simulink model "Main_Data_FlowAyush_V1"  (R2023b)
settings: Solver=FixedStepAuto  StartTime=0.0  StopTime=10.0  FixedStep=1e-3  RelTol=1e-3  EnableMultiTasking=on
undefined symbols (not defined in the file): D0, D1, D10, D11, D12, D13, D14, D15, D2, D3, D4, D5, D6, D7, D8, D9, PTA0, PTA1, PTA2, PTB23, PTB9, PTC16, PTC17, PTC2, PTC3, PTC4, PTD0, PTD1, PTD2, PTD3, PTE24, PTE25
libraries: frdmk64flib x16
settings Model: ExtModeTrigDuration=5  Creator=sadeg  LastModifiedBy=ayush
settings OptimizationCC: EnhancedBackFolding=on  PassReuseOutputArgsThreshold=0  MaxStackSize=64  OptimizeBlockOrder=speed  DifferentSizesBufferReuse=on  OptimizationCustomize=off
settings DebuggingCC: ParameterTunabilityLossMsg=error
settings HardwareCC: ProdBitPerPointer=32  ProdBitPerSizeT=32  ProdBitPerPtrDiffT=32  ProdLargestAtomicInteger=Long  ProdLargestAtomicFloat=Double  ProdWordSize=32  ProdHWDeviceType=ARM Compatible->ARM Cortex  UseEmbeddedCoderFeatures=off
settings SFSimCC: MATLABDynamicMemAlloc=off
settings RTWCC: Description=Embedded Coder  SystemTargetFile=ert.tlc  HardwareBoard=NXP FRDM-K64F  TLCOptions="-aInlineSetEventsForThisBaseRateFcn=TLC_FALSE -aSuppressMultiTaskScheduler=TLC_FALSE  -aRateBasedStepFcn=0"  TemplateMakefile=ert_default_tmf  Toolchain=GNU Tools for ARM Embedded Processors
settings CodeAppCC: ForceParamTrailComments=on  OperatorAnnotations=on
settings ERTTargetCC: ERTCustomFileBanners=off  SupportContinuousTime=on  SupportNonInlinedSFcns=on  RemoveResetFunc=off  ModelStepFunctionPrototypeControlCompliant=off  ExtModeTransport=4  ExtModeMexFile=sendToCommService

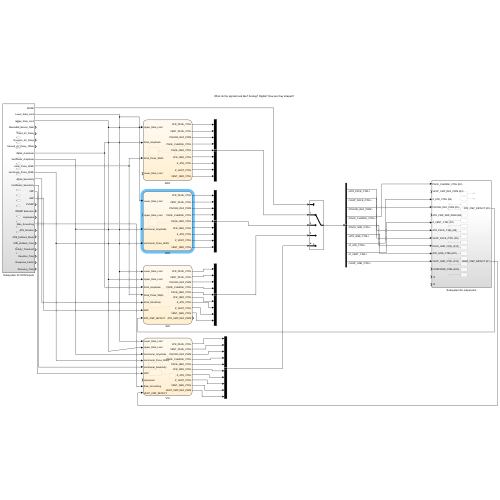
[thumbnail: Simulink's stored preview of the top-level diagram]
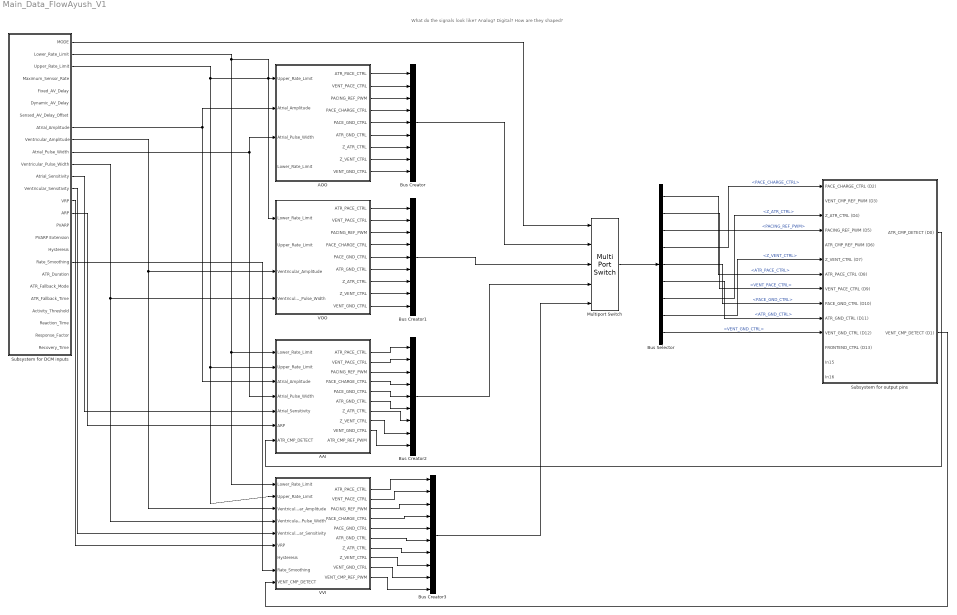
== system Main_Data_FlowAyush_V1 ==
  note: What do the signals look like? Analog? Digital? How are they shaped?
  AAI : Stateflow chart  TreatAsAtomicUnit=on
  AOO : Stateflow chart  TreatAsAtomicUnit=on
      settings: PortSchema="{\"entries\":[{\"content\":{\"sides\":[{\"content\":{\"connectorIds\":[\"In1\",\"In2\",\"In3\",\"In4\"]},\"type\":\"ConnectorPlacement.EquallySpacedRectSide\",\"uuid\":\"492a7fcf-0136-4cc6-a368-2e6eb8f4a8f6\"},{\"content\":{\"connectorIds\":[\"Out1\",\"Out2\",\"Out3\",\"Out4\",\"Out5\",\"Out8\",\"Out6\",\"Out7\",\"Out9\"],\"side\":\"RIGHT\"},\"type\":\"ConnectorPlacement.EquallySpacedRectSide\",\"uuid\":\"446f1639-51dc-43c3-8eec-8a39ae78ded7\"},{\"content\":{\"side\":\"TOP\"},\"type\":\"ConnectorPlacement.EquallySpacedRectSide\",\"uuid\":\"77fd6d12-343c-45d8-9399-9fe0379be2cf\"}]},\"type\":\"ConnectorPlacement.EquallySpacedConnector\",\"uuid\":\"42a5ffd8-4660-4821-97a9-3a811e8cbc3e\"}],\"packageUris\":[\"http://schema.mathworks.com/mf0/Connector/R2020b\"],\"version\":\"1.0\"}"
  Bus Creator : BusCreator  Inputs=9
  Bus Creator1 : BusCreator  Inputs=9
  Bus Creator2 : BusCreator  Inputs=9
  Bus Creator3 : BusCreator  Inputs=10
  Bus Selector : BusSelector  OutputSignals=ATR_PACE_CTRL,VENT_PACE_CTRL,PACING_REF_PWM,PACE_CHARGE_CTRL,PACE_GND_CTRL,ATR_GND_CTRL,Z_ATR_CTRL,Z_VENT_CTRL,VENT_GND_CTRL
  Multiport Switch : MultiPortSwitch  Inputs=4  SaturateOnIntegerOverflow=off  InputSameDT=off
  Subsystem for DCM inputs : Subsystem
  Subsystem for output pins : Subsystem
  VOO : Stateflow chart  TreatAsAtomicUnit=on
  VVI : Stateflow chart  TreatAsAtomicUnit=on
  wires:
  Subsystem for DCM inputs/2(Lower_Rate_Limit) -> VVI/1(Lower_Rate_Limit), AAI/1(Lower_Rate_Limit), VOO/1(Lower_Rate_Limit)
  Subsystem for DCM inputs/3(Upper_Rate_Limit) -> VVI/2(Upper_Rate_Limit), AAI/2(Upper_Rate_Limit), AOO/1(Upper_Rate_Limit)
  Subsystem for DCM inputs/8(Atrial_Amplitude) -> AAI/3(Atrial_Amplitude), AOO/2(Atrial_Amplitude)
  Subsystem for DCM inputs/10(Atrial_Pulse_Width) -> AAI/4(Atrial_Pulse_Width), AOO/3(Atrial_Pulse_Width)
  Subsystem for DCM inputs/9(Ventricular_Amplitude) -> VVI/3(Ventricular_Amplitude), VOO/3(Ventricular_Amplitude)
  Subsystem for DCM inputs/11(Ventricular_Pulse_Width) -> VVI/4(Ventricular_Pulse_Width), VOO/4(Ventricular_Pulse_Width)
  Subsystem for DCM inputs/12(Atrial_Sensitivity) -> AAI/5(Atrial_Sensitivity)
  Subsystem for DCM inputs/15(ARP) -> AAI/6(ARP)
  Subsystem for DCM inputs/19(Rate_Smoothing) -> VVI/8(Rate_Smoothing)
  Subsystem for DCM inputs/13(Ventricular_Sensitivity) -> VVI/5(Ventricular_Sensitivity)
  Subsystem for DCM inputs/14(VRP) -> VVI/6(VRP)
  AOO/1(ATR_PACE_CTRL) -> Bus Creator/1
  AOO/2(VENT_PACE_CTRL) -> Bus Creator/2
  AOO/3(PACING_REF_PWM) -> Bus Creator/3
  AOO/4(PACE_CHARGE_CTRL) -> Bus Creator/4
  AOO/5(PACE_GND_CTRL) -> Bus Creator/5
  AOO/8(ATR_GND_CTRL) -> Bus Creator/6
  AOO/6(Z_ATR_CTRL) -> Bus Creator/7
  AOO/7(Z_VENT_CTRL) -> Bus Creator/8
  AOO/9(VENT_GND_CTRL) -> Bus Creator/9
  VOO/1(ATR_PACE_CTRL) -> Bus Creator1/1
  VOO/2(VENT_PACE_CTRL) -> Bus Creator1/2
  VOO/3(PACING_REF_PWM) -> Bus Creator1/3
  VOO/4(PACE_CHARGE_CTRL) -> Bus Creator1/4
  VOO/5(PACE_GND_CTRL) -> Bus Creator1/5
  VOO/6(ATR_GND_CTRL) -> Bus Creator1/6
  VOO/7(Z_ATR_CTRL) -> Bus Creator1/7
  VOO/8(Z_VENT_CTRL) -> Bus Creator1/8
  VOO/9(VENT_GND_CTRL) -> Bus Creator1/9
  AAI/9(VENT_GND_CTRL) -> Bus Creator2/9
  AAI/2(VENT_PACE_CTRL) -> Bus Creator2/2
  AAI/1(ATR_PACE_CTRL) -> Bus Creator2/1
  AAI/4(PACE_CHARGE_CTRL) -> Bus Creator2/4
  AAI/6(ATR_GND_CTRL) -> Bus Creator2/6
  AAI/3(PACING_REF_PWM) -> Bus Creator2/3
  AAI/7(Z_ATR_CTRL) -> Bus Creator2/7
  AAI/8(Z_VENT_CTRL) -> Bus Creator2/8
  AAI/5(PACE_GND_CTRL) -> Bus Creator2/5
  VVI/9(VENT_GND_CTRL) -> Bus Creator3/9
  VVI/2(VENT_PACE_CTRL) -> Bus Creator3/2
  VVI/1(ATR_PACE_CTRL) -> Bus Creator3/1
  VVI/4(PACE_CHARGE_CTRL) -> Bus Creator3/4
  VVI/6(ATR_GND_CTRL) -> Bus Creator3/6
  VVI/3(PACING_REF_PWM) -> Bus Creator3/3
  VVI/7(Z_ATR_CTRL) -> Bus Creator3/7
  VVI/8(Z_VENT_CTRL) -> Bus Creator3/8
  VVI/5(PACE_GND_CTRL) -> Bus Creator3/5
  Multiport Switch/1 -> Bus Selector/1
  Bus Creator/1 -> Multiport Switch/2
  Bus Creator1/1 -> Multiport Switch/3
  Bus Creator2/1 -> Multiport Switch/4
  Bus Creator3/1 -> Multiport Switch/5
  Subsystem for DCM inputs/1(MODE) -> Multiport Switch/1
  Bus Selector/1 -> Subsystem for output pins/7(ATR_PACE_CTRL (D8))  "<ATR_PACE_CTRL>"
  Bus Selector/2 -> Subsystem for output pins/8(VENT_PACE_CTRL (D9))  "<VENT_PACE_CTRL>"
  Bus Selector/3 -> Subsystem for output pins/4(PACING_REF_PWM (D5))  "<PACING_REF_PWM>"
  Bus Selector/4 -> Subsystem for output pins/1(PACE_CHARGE_CTRL (D2))  "<PACE_CHARGE_CTRL>"
  Bus Selector/5 -> Subsystem for output pins/9(PACE_GND_CTRL (D10))  "<PACE_GND_CTRL>"
  Bus Selector/6 -> Subsystem for output pins/10(ATR_GND_CTRL (D11))  "<ATR_GND_CTRL>"
  Bus Selector/7 -> Subsystem for output pins/3(Z_ATR_CTRL (D4))  "<Z_ATR_CTRL>"
  Bus Selector/8 -> Subsystem for output pins/6(Z_VENT_CTRL (D7))  "<Z_VENT_CTRL>"
  Bus Selector/9 -> Subsystem for output pins/11(VENT_GND_CTRL (D12))  "<VENT_GND_CTRL>"
  VVI/10(VENT_CMP_REF_PWM) -> Bus Creator3/10
  Subsystem for output pins/2(VENT_CMP_DETECT (D1)) -> VVI/9(VENT_CMP_DETECT)
  Subsystem for output pins/1(ATR_CMP_DETECT (D0)) -> AAI/7(ATR_CMP_DETECT)

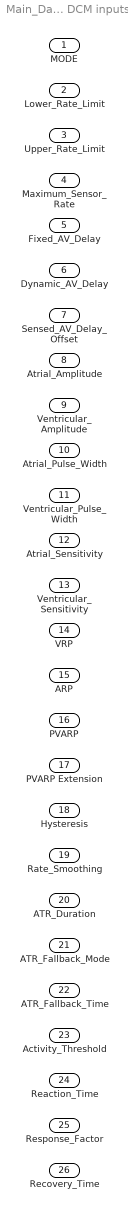
== system Main_Data_FlowAyush_V1/Subsystem for DCM inputs ==
  MODE : Outport
  Lower_Rate_Limit : Outport  Port=2
  Upper_Rate_Limit : Outport  Port=3
  Maximum_Sensor_Rate : Outport  Port=4
  Fixed_AV_Delay : Outport  Port=5
  Dynamic_AV_Delay : Outport  Port=6
  Sensed_AV_Delay_Offset : Outport  Port=7
  Atrial_Amplitude : Outport  Port=8
  Ventricular_Amplitude : Outport  Port=9
  Atrial_Pulse_Width : Outport  Port=10
  Ventricular_Pulse_Width : Outport  Port=11
  Atrial_Sensitivity : Outport  Port=12
  Ventricular_Sensitivity : Outport  Port=13
  VRP : Outport  Port=14
  ARP : Outport  Port=15
  PVARP : Outport  Port=16
  PVARP Extension : Outport  Port=17
  Hysteresis : Outport  Port=18
  Rate_Smoothing : Outport  Port=19
  ATR_Duration : Outport  Port=20
  ATR_Fallback_Mode : Outport  Port=21
  ATR_Fallback_Time : Outport  Port=22
  Activity_Threshold : Outport  Port=23
  Reaction_Time : Outport  Port=24
  Response_Factor : Outport  Port=25
  Recovery_Time : Outport  Port=26

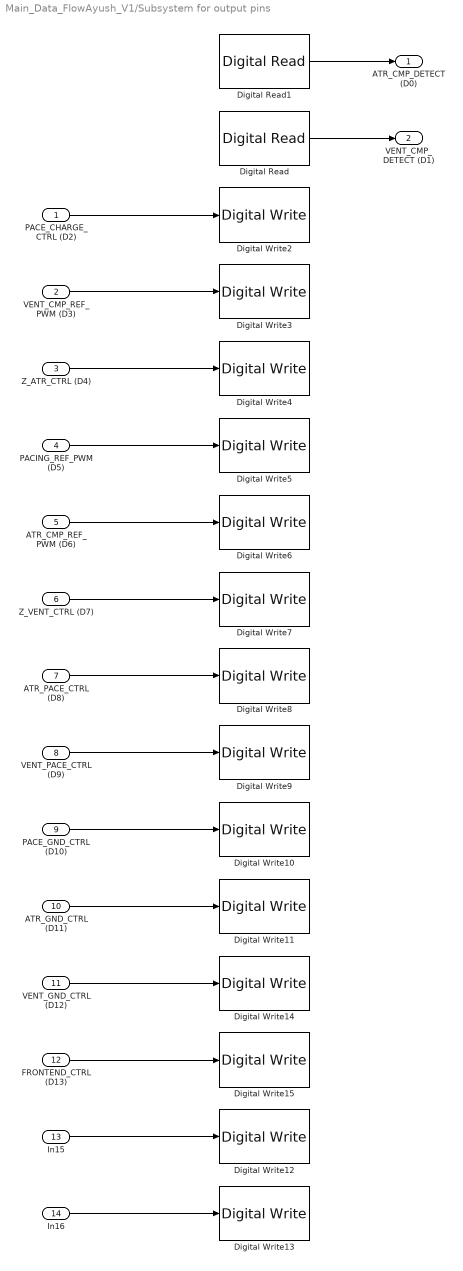
== system Main_Data_FlowAyush_V1/Subsystem for output pins ==
  PACE_CHARGE_CTRL (D2) : Inport
  VENT_CMP_REF_PWM (D3) : Inport  Port=2
  Z_ATR_CTRL (D4) : Inport  Port=3
  PACING_REF_PWM (D5) : Inport  Port=4
  ATR_CMP_REF_PWM (D6) : Inport  Port=5
  Z_VENT_CTRL (D7) : Inport  Port=6
  ATR_PACE_CTRL (D8) : Inport  Port=7
  VENT_PACE_CTRL (D9) : Inport  Port=8
  PACE_GND_CTRL (D10) : Inport  Port=9
  ATR_GND_CTRL (D11) : Inport  Port=10
  VENT_GND_CTRL (D12) : Inport  Port=11
  FRONTEND_CTRL (D13) : Inport  Port=12
  In15 : Inport  Port=13
  In16 : Inport  Port=14
  Digital Read : frdmk64flib/Digital Read  Whichpin=PTC17 (D1)  SampleTime=-1
  Digital Read1 : frdmk64flib/Digital Read  Whichpin=PTC16 (D0)  SampleTime=-1
  Digital Write10 : frdmk64flib/Digital Write  Whichpin=PTD0 (D10)
  Digital Write11 : frdmk64flib/Digital Write  Whichpin=PTD2 (D11)
  Digital Write12 : frdmk64flib/Digital Write  Whichpin=PTE25 (D14)
  Digital Write13 : frdmk64flib/Digital Write  Whichpin=PTE24 (D15)
  Digital Write14 : frdmk64flib/Digital Write  Whichpin=PTD3 (D12)
  Digital Write15 : frdmk64flib/Digital Write  Whichpin=PTD1 (D13)
  Digital Write2 : frdmk64flib/Digital Write  Whichpin=PTB9 (D2)
  Digital Write3 : frdmk64flib/Digital Write  Whichpin=PTA1 (D3)
  Digital Write4 : frdmk64flib/Digital Write  Whichpin=PTB23 (D4)
  Digital Write5 : frdmk64flib/Digital Write  Whichpin=PTA2 (D5)
  Digital Write6 : frdmk64flib/Digital Write  Whichpin=PTC2 (D6)
  Digital Write7 : frdmk64flib/Digital Write  Whichpin=PTC3 (D7)
  Digital Write8 : frdmk64flib/Digital Write  Whichpin=PTA0 (D8)
  Digital Write9 : frdmk64flib/Digital Write  Whichpin=PTC4 (D9)
  ATR_CMP_DETECT (D0) : Outport
  VENT_CMP_DETECT (D1) : Outport  Port=2
  wires:
  PACE_CHARGE_CTRL (D2)/1 -> Digital Write2/1
  Z_ATR_CTRL (D4)/1 -> Digital Write4/1
  VENT_CMP_REF_PWM (D3)/1 -> Digital Write3/1
  PACING_REF_PWM (D5)/1 -> Digital Write5/1
  Z_VENT_CTRL (D7)/1 -> Digital Write7/1
  ATR_CMP_REF_PWM (D6)/1 -> Digital Write6/1
  PACE_GND_CTRL (D10)/1 -> Digital Write10/1
  ATR_GND_CTRL (D11)/1 -> Digital Write11/1
  ATR_PACE_CTRL (D8)/1 -> Digital Write8/1
  VENT_PACE_CTRL (D9)/1 -> Digital Write9/1
  In15/1 -> Digital Write12/1
  VENT_GND_CTRL (D12)/1 -> Digital Write14/1
  FRONTEND_CTRL (D13)/1 -> Digital Write15/1
  In16/1 -> Digital Write13/1
  Digital Read/1 -> VENT_CMP_DETECT (D1)/1
  Digital Read1/1 -> ATR_CMP_DETECT (D0)/1

== stateflow chart Main_Data_FlowAyush_V1/AOO ==
  note: AOO: Pace Atrium at constant rate
  state DISCHARGE
    during:
    %Discharge C22 into Atrium
    %Begin Charging C21 Blocking Capacitor
    PACE_CHARGE_CTRL = 0;
    PACE_GND_CTRL = 1;
    ATR_PACE_CTRL = 1;
    ATR_GND_CTRL = 0;
    Z_ATR_CTRL = 0;
    Z_VENT_CTRL = 0;
    VENT_GND_CTRL = 0;
    VENT_PACE_CTRL  = 0;
  state CHARGE
    during:
    % Start Charging C22
    ATR_PACE_CTRL = 0;
    VENT_PACE_CTRL = 0;
    PACING_REF_PWM = Atrial_Amplitude
    PACE_CHARGE_CTRL = 1;
    %Begin Discharging C21 Blocking Capacitor
    PACE_GND_CTRL = 1;
    VENT_PACE_CTRL = 0;
    VENT_GND_CTRL = 0;
    Z_ATR_CTRL = 0;
    Z_VENT_CTRL = 0;
    ATR_PACE_CTRL = 0;
    ATR_GND_CTRL = 1;
  (default) -> CHARGE
  CHARGE -> DISCHARGE : after((60/Lower_Rate_Limit) - (Atrial_Pulse_Width/1000), sec)
  DISCHARGE -> CHARGE : after({Atrial_Pulse_Width},msec)
  data: Upper_Rate_Limit input; Atrial_Amplitude input; Atrial_Pulse_Width input; ATR_PACE_CTRL output; VENT_PACE_CTRL output; PACING_REF_PWM output; PACE_CHARGE_CTRL output; PACE_GND_CTRL output; Z_ATR_CTRL output; Z_VENT_CTRL output; ATR_GND_CTRL output; VENT_GND_CTRL output; Lower_Rate_Limit input

== stateflow chart Main_Data_FlowAyush_V1/VVI ==
  state hold
    entry:
  note: skip pulse if natural heart beat is detected
  state PULSE_VENT
    entry:
    PACE_CHARGE_CTRL = 0;
    VENT_GND_CTRL = 0;
    VENT_PACE_CTRL = 1;
  state CHARGE
    entry:
    VENT_PACE_CTRL = 0;
    PACE_CHARGE_CTRL = 1;
  state INIT
    entry:
    VENT_CMP_REF_PWM = Ventricular_Sensitivity;
    PACING_REF_PWM = Ventricular_Amplitude;
    VENT_GND_CTRL = 0;
    VENT_PACE_CTRL = 0;
    Z_ATR_CTRL = 0;
    Z_VENT_CTRL = 0;
    PACE_GND_CTRL = 1;
  state DISCHARGE
    entry:
    VENT_PACE_CTRL = 0;
    VENT_GND_CTRL = 1;
  hold -> PULSE_VENT [order 1] : after((60000/Lower_Rate_Limit) - Ventricular_Pulse_Width+VRP, msec)
  CHARGE -> hold : after(VRP, msec)
  hold -> CHARGE [order 2] : [VENT_CMP_DETECT == 1]
  INIT -> CHARGE
  PULSE_VENT -> DISCHARGE : after(Ventricular_Pulse_Width, msec)
  (default) -> INIT
  DISCHARGE -> INIT
  data: Lower_Rate_Limit input; Upper_Rate_Limit input; Ventricular_Amplitude input; Ventricular_Pulse_Width input; Ventricular_Sensitivity input; VRP input; Hysteresis input; Rate_Smoothing input; ATR_PACE_CTRL output; VENT_PACE_CTRL output; PACING_REF_PWM output; PACE_CHARGE_CTRL output; PACE_GND_CTRL output; ATR_GND_CTRL output; Z_ATR_CTRL output; Z_VENT_CTRL output; VENT_GND_CTRL output; VENT_CMP_REF_PWM output; VENT_CMP_DETECT input

== stateflow chart Main_Data_FlowAyush_V1/VOO ==
  note: VOO: Pace Ventrical at constant rate
  state DISCHARGE
    during:
    %Discharge C22 into Ventrical
    %Begin Charging C21 Blocking Capacitor
    PACE_CHARGE_CTRL = 0;
    PACE_GND_CTRL = 1;
    ATR_PACE_CTRL = 0;
    ATR_GND_CTRL = 0;
    Z_ATR_CTRL = 0;
    Z_VENT_CTRL = 0;
    VENT_GND_CTRL = 0;
    VENT_PACE_CTRL  = 1;
  state CHARGE
    during:
    % Start Charging C22
    ATR_PACE_CTRL = 0;
    VENT_PACE_CTRL = 0;
    PACING_REF_PWM = Ventricular_Amplitude
    PACE_CHARGE_CTRL = 1;
    %Begin Discharging C21 Blocking Capacitor
    PACE_GND_CTRL = 1;
    VENT_PACE_CTRL = 0;
    VENT_GND_CTRL = 0;
    Z_ATR_CTRL = 0;
    Z_VENT_CTRL = 0;
    ATR_PACE_CTRL = 0;
    ATR_GND_CTRL = 1;
  (default) -> CHARGE
  CHARGE -> DISCHARGE : after((60/Lower_Rate_Limit) - (Ventricular_Pulse_Width/1000), sec)
  DISCHARGE -> CHARGE : after({Ventricular_Pulse_Width})
  data: Lower_Rate_Limit input; Upper_Rate_Limit input; Ventricular_Amplitude input; Ventricular_Pulse_Width input; ATR_PACE_CTRL output; VENT_PACE_CTRL output; PACING_REF_PWM output; PACE_CHARGE_CTRL output; PACE_GND_CTRL output; ATR_GND_CTRL output; Z_ATR_CTRL output; Z_VENT_CTRL output; VENT_GND_CTRL output

== stateflow chart Main_Data_FlowAyush_V1/AAI ==
  note: AAI will only pace the atrium if the natural heartbeat drops below that of the defined lower limit
  state hold
    entry:
  note: skip pulse if natural heart beat is detected
  state PULSE_ATR
    entry:
    PACE_CHARGE_CTRL = 0;
    ATR_GND_CTRL = 0;
    ATR_PACE_CTRL = 1;
  state CHARGE
    entry:
    ATR_PACE_CTRL = 0;
    PACE_CHARGE_CTRL = 1;
  state INIT
    entry:
    ATR_CMP_REF_PWM = Atrial_Sensitivity;
    PACING_REF_PWM = Atrial_Amplitude;
    VENT_GND_CTRL = 0;
    VENT_PACE_CTRL = 0;
    Z_ATR_CTRL = 0;
    Z_VENT_CTRL = 0;
    PACE_GND_CTRL = 1;
  state DISCHARGE
    entry:
    ATR_PACE_CTRL = 0;
    ATR_GND_CTRL = 1;
  hold -> PULSE_ATR [order 1] : after((60000/Lower_Rate_Limit) - (Atrial_Pulse_Width)+ARP, msec)
  CHARGE -> hold : after(ARP, msec)
  hold -> CHARGE [order 2] : [ATR_CMP_DETECT == 1]
  INIT -> CHARGE
  PULSE_ATR -> DISCHARGE : after(Atrial_Pulse_Width, msec)
  (default) -> INIT
  DISCHARGE -> INIT
  data: Lower_Rate_Limit input; Upper_Rate_Limit input; Atrial_Amplitude input; Atrial_Pulse_Width input; Atrial_Sensitivity input; ARP input; ATR_PACE_CTRL output; VENT_PACE_CTRL output; PACING_REF_PWM output; PACE_CHARGE_CTRL output; PACE_GND_CTRL output; ATR_GND_CTRL output; Z_ATR_CTRL output; Z_VENT_CTRL output; VENT_GND_CTRL output; ATR_CMP_DETECT input; ATR_CMP_REF_PWM output
